simulink model "sim_sil_test"  (Simulink 8.1)
settings: Solver=FixedStepDiscrete  StartTime=0.0  StopTime=100.0  FixedStep=T  RelTol=1e-3
PostLoadFcn:
  | sim_test_data
StartFcn:
  | sim_test_data
values from neighbouring files (symbols this model uses):
  T = 1    [sim_test_data.m]
settings Model: Creator=evarshavskaya  LastModifiedBy=evarshavskaya
settings DataIOCC: ExternalInput=off  InitialState=off  LimitDataPoints=off  SaveOutput=off  SignalLogging=off  SaveTime=off
settings OptimizationCC: InlineParams=on  OptimizeModelRefInitCode=on  LifeSpan=1
settings DebuggingCC: InheritedTsInSrcMsg=none  SingleTaskRateTransMsg=error  UnconnectedInputMsg=error  UnconnectedOutputMsg=error  UnconnectedLineMsg=error  UnknownTsInhSupMsg=error
settings HardwareCC: ProdIntDivRoundTo=Zero  ProdEndianess=LittleEndian  ProdHWDeviceType=Generic->Custom
settings RTWCC: SystemTargetFile=ert.tlc  TemplateMakefile=ert_default_tmf  PostCodeGenCommand=rappid_analyzegencode(buildInfo)  Description=Embedded Coder  ProcessScript=ert_make_rtw_hook  PortableWordSizes=on
settings CodeAppCC: IgnoreCustomStorageClasses=off  MaxIdLength=63  CustomSymbolStrType=$N$R$M  InternalIdentifier=Classic
settings ERTTargetCC: CodeReplacementLibrary=ANSI_C  MultiwordLength=2048  GenerateSampleERTMain=on  InlinedParameterPlacement=NonHierarchical  ERTCustomFileTemplate=example_file_process.tlc  ConvertIfToSwitch=off  SuppressUnreachableDefaultCases=off

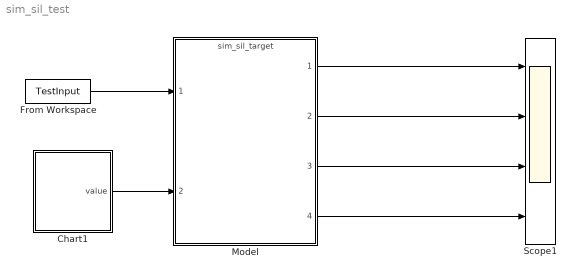
== system sim_sil_test ==
  Chart1 : Stateflow chart  TreatAsAtomicUnit=on
  From Workspace : FromWorkspace  VariableName=TestInput  SampleTime=T
  Model : ModelReference  ModelNameDialog=sim_sil_target  SimulationMode=Software-in-the-loop (SIL)  ModelReferenceVersion=1.142  CopyOfModelName=sim_sil_target  DefaultDataLogging=off
  Scope1 : Scope  NumInputPorts=4
      settings: TimeRange=100  YMin=5000~-1~0~0  YMax=30000~1~1~1
  wires:
  From Workspace/1 -> Model/1
  Model/1 -> Scope1/1
  Model/2 -> Scope1/2
  Model/3 -> Scope1/3
  Model/4 -> Scope1/4
  Chart1/1(value) -> Model/2

== stateflow chart Chart1 ==
  settings: executeAtInitialization=1
  state A
    du:
    cntr=cntr+0.2;
    value=cntr;
    ex:
    cntr = -3.14;
  (default) -> A : {cntr=0;}
  A -> A : [cntr >= 3.14]
  data: cntr local single =0; value output single
